simulink model "SLIPrun"  (R2015a)
settings: Solver=ode45  StartTime=0.0  StopTime=5  MaxStep=0.01  RelTol=1e-3
InitFcn:
  | SLIPrun_params
values from neighbouring files (symbols this model uses):
  dx0 = 0.4138    [SLIPquad_params.m]    (also in SLIPrun_params.m = 3; SLIPwalk_params.m = 2.5; smm_params.m = 5)
  dy0 = 0.1683    [SLIPquad_params.m]    (also in SLIPrun_params.m = -1; SLIPwalk_params.m = 0; smm_params.m = 0)
  g = 1    [SLIPquad_params.m]    (also in SLIPrun_params.m = 9.81; SLIPwalk_params.m = 9.81; smm_params.m = 9.81)
  k = 20    [SLIPquad_params.m]    (also in SLIPrun_params.m = 23000; SLIPwalk_params.m = 10000; smm_params.m = 20000)
  kv = 0    [SLIPrun_params.m]    (also in SLIPwalk_params.m = 100000)
  l0 = 1    [SLIPquad_params.m]    (also in SLIPrun_params.m; SLIPwalk_params.m; smm_params.m)
  m = 1    [SLIPquad_params.m]    (also in SLIPrun_params.m = 70; SLIPwalk_params.m = 70; smm_params.m = 80)
  theta_th = 15*pi/180    (= 0.261799387799)    [SLIPrun_params.m]    (also in SLIPwalk_params.m = 0.349065850399)
  x0 = []    [AnimQUAD.m]    (also in AnimQUAD2.m; AnimSMR.m; SLIPquad_params.m = 0; SLIPrun_params.m = -l*sin(theta_th))
  y0 = 1.0237    [SLIPquad_params.m]    (also in SLIPrun_params.m = sqrt(l^2 - x0^2); SLIPwalk_params.m = sqrt(l0^2 - x0^2); smm_params.m = 1)
libraries: simulink_extras x1
settings Model: CovSFcnEnable=off  Creator=Joe  LastModifiedBy=Joe
settings DebuggingCC: SolverPrmCheckMsg=warning

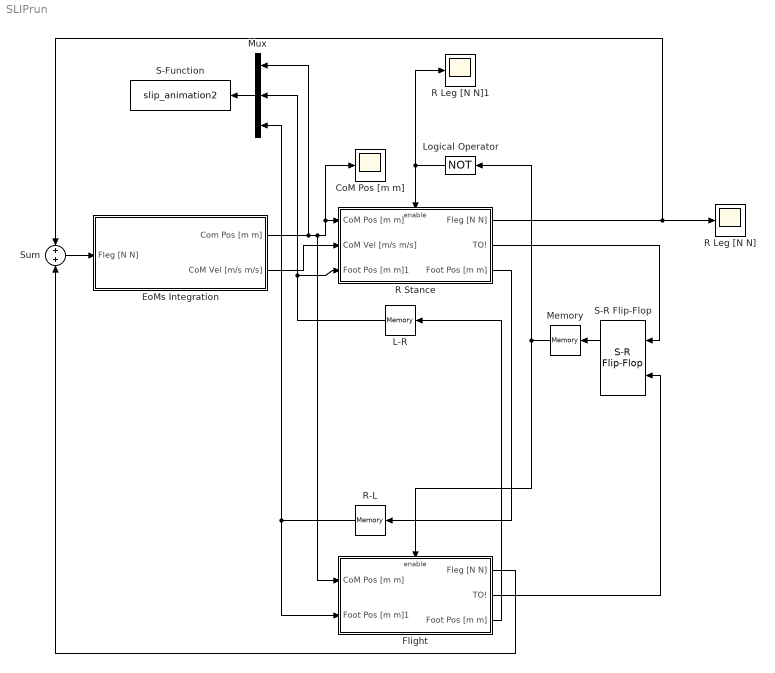
== system SLIPrun ==
  CoM Pos [m m] : Scope
      settings: YMin=0  YMax=1
  EoMs Integration : Subsystem
  Flight : Subsystem
  L-R : Memory
  Logical Operator : Logic  Operator=NOT  AllPortsSameDT=off  OutDataTypeStr=boolean
  Memory : Memory
  Mux : Mux  Inputs=3
  R Leg [N N] : Scope
      settings: YMin=-500  YMax=2750  SaveName=ScopeData2
  R Leg [N N]1 : Scope
      settings: SaveName=ScopeData3
  R Stance : Subsystem
  R-L : Memory
  S-Function : S-Function  FunctionName=slip_animation2  Parameters=0.001
  S-R Flip-Flop : simulink_extras/Flip Flops/S-R Flip-Flop  initial_condition=0
  Sum : Sum
  wires:
  EoMs Integration/2(CoM Vel [m/s m/s]) -> R Stance/2(CoM Vel [m/s m/s])
  R Stance/1(Fleg [N N]) -> Sum/1, R Leg [N N]/1
  Logical Operator/1 -> R Stance/Enable, R Leg [N N]1/1
  R Stance/3(Foot Pos [m m]) -> R-L/1
  R-L/1 -> Flight/2(Foot Pos [m m]1), Mux/3
  Flight/1(Fleg [N N]) -> Sum/2
  Sum/1 -> EoMs Integration/1(Fleg [N N])
  Mux/1 -> S-Function/1
  EoMs Integration/1(Com Pos [m m]) -> Mux/1, Flight/1(CoM Pos [m m]), CoM Pos [m m]/1, R Stance/1(CoM Pos [m m])
  Flight/3(Foot Pos [m m]) -> L-R/1
  L-R/1 -> Mux/2, R Stance/3(Foot Pos [m m]1)
  R Stance/2(TO!) -> S-R Flip-Flop/1
  Flight/2(TO!) -> S-R Flip-Flop/2
  S-R Flip-Flop/1 -> Memory/1
  Memory/1 -> Flight/Enable, Logical Operator/1

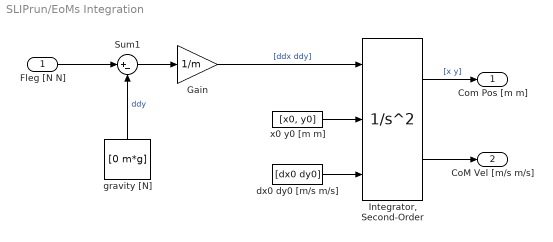
== system SLIPrun/EoMs Integration ==
  Fleg [N N] : Inport
  Gain : Gain  Gain=1/m
  "Integrator, Second-Order" : SecondOrderIntegrator  ICSourceX=external  ICSourceDXDT=external
  Sum1 : Sum  Inputs=|+-
  dx0 dy0 [m/s m/s] : Constant  Value=[dx0 dy0]
  gravity [N] : Constant  Value=[0 m*g]
  x0 y0 [m m] : Constant  Value=[x0, y0]
  Com Pos [m m] : Outport
  CoM Vel [m/s m/s] : Outport  Port=2
  wires:
  Gain/1 -> "Integrator, Second-Order"/1  "[ddx ddy]"
  Fleg [N N]/1 -> Sum1/1
  x0 y0 [m m]/1 -> "Integrator, Second-Order"/2
  dx0 dy0 [m/s m/s]/1 -> "Integrator, Second-Order"/3
  gravity [N]/1 -> Sum1/2  "ddy"
  "Integrator, Second-Order"/1 -> Com Pos [m m]/1  "[x y]"
  Sum1/1 -> Gain/1
  "Integrator, Second-Order"/2 -> CoM Vel [m/s m/s]/1

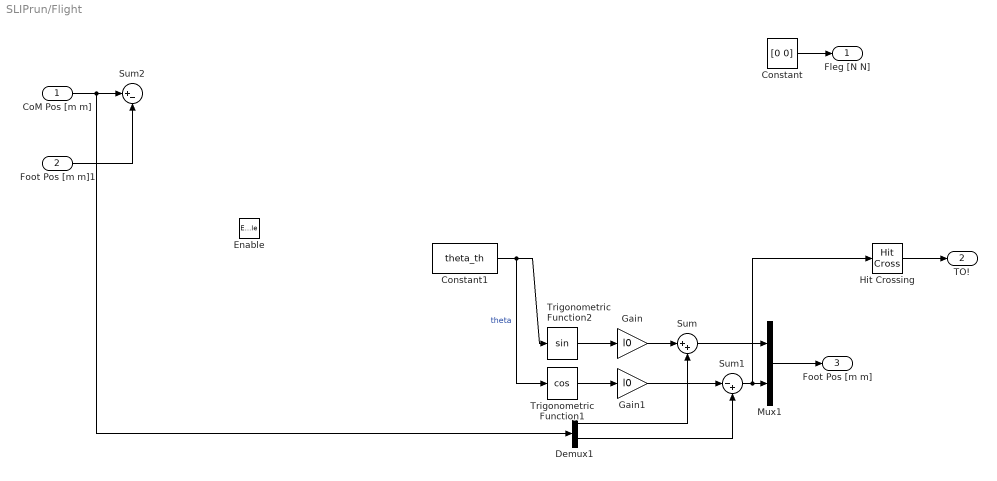
== system SLIPrun/Flight ==
  CoM Pos [m m] : Inport
  Foot Pos [m m]1 : Inport  Port=2
  Enable : EnablePort  StatesWhenEnabling=reset
  Constant : Constant  Value=[0 0]
  Constant1 : Constant  Value=theta_th
  Demux1 : Demux  Outputs=2
  Gain : Gain  Gain=l0
  Gain1 : Gain  Gain=l0
  Hit Crossing : HitCross  HitCrossingDirection=falling
  Mux1 : Mux  Inputs=2
  Sum : Sum  Inputs=|++
  Sum1 : Sum  Inputs=|-+
  Sum2 : Sum  Inputs=|+-
  Trigonometric Function1 : Trigonometry  Operator=cos
  Trigonometric Function2 : Trigonometry
  Fleg [N N] : Outport  OutputWhenDisabled=reset  InitialOutput=[0 0]
  TO! : Outport  Port=2  OutputWhenDisabled=reset  InitialOutput=[0]
  Foot Pos [m m] : Outport  Port=3
  wires:
  Constant/1 -> Fleg [N N]/1
  Constant1/1 -> Trigonometric Function1/1, Trigonometric Function2/1  "theta"
  Trigonometric Function2/1 -> Gain/1
  Trigonometric Function1/1 -> Gain1/1
  Gain1/1 -> Sum1/1
  Gain/1 -> Sum/1
  Demux1/1 -> Sum/2
  Demux1/2 -> Sum1/2
  Sum1/1 -> Hit Crossing/1, Mux1/2
  Sum/1 -> Mux1/1
  Mux1/1 -> Foot Pos [m m]/1
  CoM Pos [m m]/1 -> Demux1/1, Sum2/1
  Foot Pos [m m]1/1 -> Sum2/2
  Hit Crossing/1 -> TO!/1

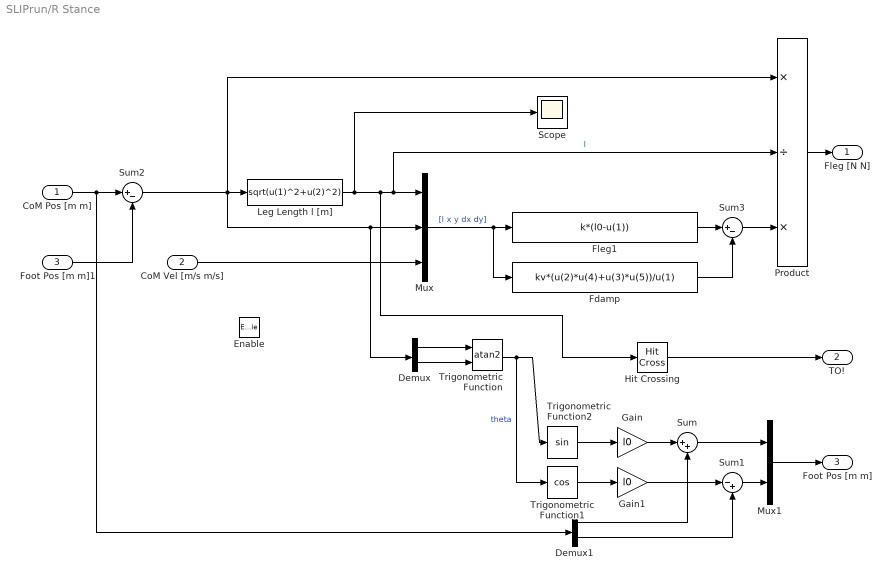
== system SLIPrun/R Stance ==
  CoM Pos [m m] : Inport
  CoM Vel [m/s m/s] : Inport  Port=2
  Foot Pos [m m]1 : Inport  Port=3
  Enable : EnablePort  StatesWhenEnabling=reset
  Demux : Demux  Outputs=2
  Demux1 : Demux  Outputs=2
  Fdamp : Fcn  Expr=kv*(u(2)*u(4)+u(3)*u(5))/u(1)
  Fleg1 : Fcn  Expr=k*(l0-u(1))
  Gain : Gain  Gain=l0
  Gain1 : Gain  Gain=l0
  Hit Crossing : HitCross  HitCrossingOffset=l0  HitCrossingDirection=rising
  Leg Length l [m] : Fcn  Expr=sqrt(u(1)^2+u(2)^2)
  Mux : Mux  Inputs=3
  Mux1 : Mux  Inputs=2
  Product : Product  Inputs=*/*
  Scope : Scope
      settings: YMin=0.85  YMax=1.025
  Sum : Sum  Inputs=|++
  Sum1 : Sum  Inputs=|-+
  Sum2 : Sum  Inputs=|+-
  Sum3 : Sum  Inputs=|+-
  Trigonometric Function : Trigonometry  Operator=atan2
  Trigonometric Function1 : Trigonometry  Operator=cos
  Trigonometric Function2 : Trigonometry
  Fleg [N N] : Outport  OutputWhenDisabled=reset  InitialOutput=[0 0]
  TO! : Outport  Port=2  OutputWhenDisabled=reset  InitialOutput=[0]
  Foot Pos [m m] : Outport  Port=3
  wires:
  Sum2/1 -> Demux/1, Mux/2, Product/1, Leg Length l [m]/1
  Leg Length l [m]/1 -> Scope/1, Hit Crossing/1, Product/2, Mux/1  "l"
  CoM Vel [m/s m/s]/1 -> Mux/3
  Mux/1 -> Fleg1/1, Fdamp/1  "[l x y dx dy]"
  Fleg1/1 -> Sum3/1
  Product/1 -> Fleg [N N]/1
  Trigonometric Function/1 -> Trigonometric Function1/1, Trigonometric Function2/1  "theta"
  Hit Crossing/1 -> TO!/1
  Trigonometric Function2/1 -> Gain/1
  Trigonometric Function1/1 -> Gain1/1
  Gain1/1 -> Sum1/1
  Gain/1 -> Sum/1
  Demux1/1 -> Sum/2
  Demux1/2 -> Sum1/2
  Sum1/1 -> Mux1/2
  Sum/1 -> Mux1/1
  Mux1/1 -> Foot Pos [m m]/1
  CoM Pos [m m]/1 -> Demux1/1, Sum2/1
  Foot Pos [m m]1/1 -> Sum2/2
  Sum3/1 -> Product/3
  Fdamp/1 -> Sum3/2
  Demux/1 -> Trigonometric Function/1
  Demux/2 -> Trigonometric Function/2
